simulink library "cgeqlib"  (Simulink 5.0)
libraries: simulink x2
settings Model: Creator=rlang  LastModifiedBy=ralcock  ExtModeMexFile=rti_comm  RTWMakeCommand=make_rti  RTWRetainRTWFile=on

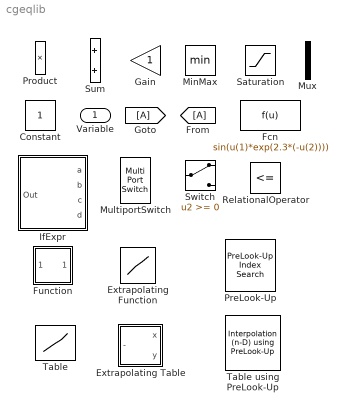
== system cgeqlib ==
  Variable : Inport  Orientation=left
      settings: OpenFcn=web(['file:///', which('block_ref.htm')]);
  Constant : Constant  Orientation=left
  Extrapolating Function : Lookup  Tag=lookupone  Orientation=left  InputValues=[-5:5]  OutputValues=tanh([-5:5])  SaturateOnIntegerOverflow=on
  Extrapolating Table : Subsystem  Tag=lookuptwo  Orientation=left  mask(Lookup Table (2-D)){x=[1:3], y=[1:3], t=[4 5 6;16 19 20;10 18 23]}
      mask prompts: x "Row:"; y "Column:"; t "Table:"
      mask help: Performs 2-D linear interpolation of input values using the specified input/output table.
      mask init:
      | [r,c]=size(t);
      | xt=reshape(x,prod(size(x)),1);
      | xi=xt(:,ones(1,c));
      | minx=min(x); maxx=max(x);
      | miny=min(y);maxy=max(y);
      | mint=min(min(t)); maxt=max(max(t));
      mask Display: plot(xi,t,[minx maxx],[mint mint],[minx minx],[mint maxt],maxx+1,maxt)
  Fcn : Fcn  Orientation=left  Expr=sin(u(1)*exp(2.3*(-u(2))))
  Function : Subsystem  Orientation=left  mask(Lookup Table (1-D)){InputValues=, OutputValues=}
      mask prompts: InputValues "Input:"; OutputValues "Output:"
      mask init:
      | if isempty(InputValues) | isempty(OutputValues)
      | minx = -1;maxx = 1;miny=-1;maxy = 1;
      | else
      | minx=min(InputValues); maxx=max(InputValues);
      | miny=min(OutputValues);maxy=max(OutputValues);
      | if minx>0;minx=0;end
      | if miny>0;miny=0;end
      | if maxx<0;maxx=0;end
      | if maxy<0;maxy=0;end
      | end
      mask Display: plot(InputValues',OutputValues',[minx; maxx],[0; 0],[0;0],[miny;maxy])
  Gain : Gain  Orientation=left  SaturateOnIntegerOverflow=on
  IfExpr : Subsystem  Tag=ifexpr  Orientation=left
      settings: OpenFcn=web(['file:///', which('block_ref.htm')]);
      mask Display: disp('IF (a<b)\n   out=c;\nELSE\n   out=d;\nEND')
  MinMax : MinMax  Orientation=left  SaturateOnIntegerOverflow=on  InputSameDT=on
  MultiportSwitch : MultiPortSwitch  Orientation=left  Inputs=3  SaturateOnIntegerOverflow=on  InputSameDT=on
  Mux : Mux  Orientation=left  Inputs=2
  PreLook-Up : simulink/Look-Up Tables/PreLook-Up Index Search  Orientation=left  bpData=[10:10:100]  searchMode=Binary Search  cacheBpFlag=off  outputFlag=off  extrapMode=Linear Extrapolation  rangeErrorMode=None
  Product : Product  Orientation=left  SaturateOnIntegerOverflow=on  InputSameDT=on
  RelationalOperator : RelationalOperator  Orientation=left  Operator=<=  InputSameDT=on
  Saturation : Saturate  Orientation=left
  Sum : Sum  Orientation=left  SaturateOnIntegerOverflow=on  InputSameDT=on
  Switch : Switch  Orientation=left  SaturateOnIntegerOverflow=on  InputSameDT=on
  Table : Lookup2D  Orientation=left  RowIndex=[1:3]  ColumnIndex=[1:3]  OutputValues=[4 5 6;16 19 20;10 18 23]  SaturateOnIntegerOverflow=on
  Table using PreLook-Up : simulink/Look-Up Tables/Interpolation (n-D) using PreLook-Up  Orientation=left  numDimsPopupSelect=2  explicitNumDims=2  table=sqrt([1:10]'*[1:10])  interpMethod=Linear  extrapMethod=Linear  rangeErrorMode=None

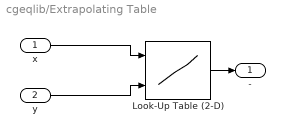
== system cgeqlib/Extrapolating Table ==
  x : Inport
  y : Inport  Port=2
  Look-Up Table (2-D) : Lookup2D  RowIndex=x  ColumnIndex=y  OutputValues=t  SaturateOnIntegerOverflow=on  InputSameDT=on
  - : Outport
  wires:
  Look-Up Table (2-D)/1 -> -/1
  x/1 -> Look-Up Table (2-D)/1
  y/1 -> Look-Up Table (2-D)/2

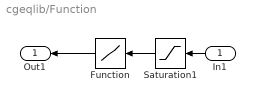
== system cgeqlib/Function ==
  In1 : Inport  Orientation=left
  Function : Lookup  Tag=lookupone  Orientation=left  InputValues=InputValues  OutputValues=OutputValues  SaturateOnIntegerOverflow=on
  Saturation1 : Saturate  Orientation=left  UpperLimit=maxx  LowerLimit=minx
  Out1 : Outport  Orientation=left
  wires:
  Function/1 -> Out1/1
  In1/1 -> Saturation1/1
  Saturation1/1 -> Function/1

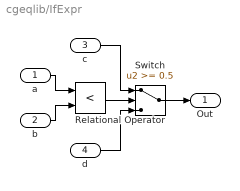
== system cgeqlib/IfExpr ==
  a : Inport
  b : Inport  Port=2
  c : Inport  Port=3
  d : Inport  Port=4
  Relational Operator : RelationalOperator  Operator=<  InputSameDT=on
  Switch : Switch  Threshold=0.5  SaturateOnIntegerOverflow=on  InputSameDT=on
  Out : Outport
  wires:
  Relational Operator/1 -> Switch/2
  c/1 -> Switch/1
  a/1 -> Relational Operator/1
  Switch/1 -> Out/1
  b/1 -> Relational Operator/2
  d/1 -> Switch/3
